simulink model "Kalman_filter"  (R2025b)
settings: Solver=FixedStepAuto  StartTime=0.0  StopTime=20  FixedStep=0.002  RelTol=1e-3
values from neighbouring files (symbols this model uses):
  A_pitch = [X_hat_u  X_hat_q   g  0 ... (first row only)    [Parameters.m]
  A_py = blkdiag(A_pitch, A_yaw)    [Parameters.m]
  A_yaw = [N_hat_r  1/I_zz ... (first row only)    [Parameters.m]
  B_py = blkdiag(B_pitch, B_yaw)    [Parameters.m]
  C_pitch = [X_hat_u+d_new*M_hat_u  X_hat_q+d_new*M_hat_q   0   d_new/I_yy;      0        1           0   0]    [Parameters.m]
  C_py = blkdiag(C_pitch, C_yaw)    [Parameters.m]
  C_yaw = [1   0]    [Parameters.m]
  k_r = 0.8e-5    (= 8e-06)    [Parameters.m]
  kd_p = 0.27*kth_p    (= 0.0005184)    [Parameters.m]
  kth_p = 192e-5    (= 0.00192)    [Parameters.m]
  L_ob_py = X1_py*C_py'*(R_n_py^-1)    [Parameters.m]
  LC_DEN = [1 p1]    [Parameters.m]
  LC_NUM = gain*(p1/z1)*[1 z1]    [Parameters.m]
  T_psi = 0.15    [Parameters.m]
  u_gain = -X_hat_u/g    (= 0.0967315158219)    [Parameters.m]
  x_hat_py = [0 0 0 0 0 0]'    [Parameters.m]
  x_pitch = [0.1 0 2*pi/180 0]'    [Parameters.m]
  x_yaw = [5*pi/180 2*pi/180 0]'    [Parameters.m]
libraries: slpidlib x2
settings Model: Creator=yfari  LastModifiedBy=yfari
settings OptimizationCC: ReuseModelBlockBuffer=off
settings DebuggingCC: UnconnectedInputMsg=warning  UnconnectedOutputMsg=warning  UnconnectedLineMsg=warning
settings ModelReferenceCC: EnableRefExpFcnMdlSchedulingChecks=on
settings RTWCC: GPUComputeCapability=3.5  DLArmComputeVersion=19.05

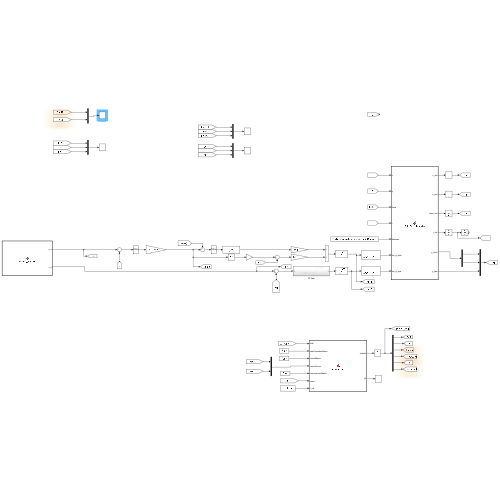
[thumbnail: Simulink's stored preview of the top-level diagram]
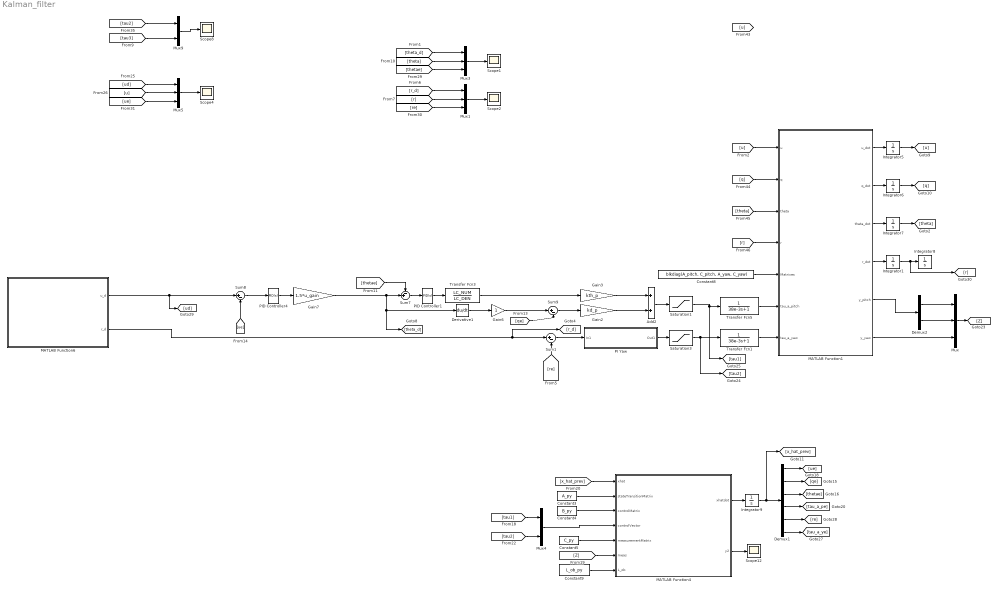
== system Kalman_filter ==
  Add2 : Sum
  Constant3 : Constant  Value=A_py
  Constant4 : Constant  Value=B_py
  Constant5 : Constant  Value=C_py
  Constant8 : Constant  Value=blkdiag(A_pitch, C_pitch, A_yaw, C_yaw)  VectorParams1D=off
  Constant9 : Constant  Value=L_ob_py
  Demux1 : Demux  Outputs=6
  Demux2 : Demux  Outputs=2
  Derivative1 : Derivative
  Gain2 : Gain  Gain=kd_p
  Gain3 : Gain  Gain=kth_p
  Gain6 : Gain
  Gain7 : Gain  Gain=1.5*u_gain
  Integrator1 : Integrator  InitialCondition=x_yaw(1)
  Integrator5 : Integrator  InitialCondition=x_pitch(1)
  Integrator6 : Integrator  InitialCondition=x_pitch(2)
  Integrator7 : Integrator  InitialCondition=x_pitch(3)
  Integrator8 : Integrator  InitialCondition=0*pi/180
  Integrator9 : Integrator  InitialCondition=x_hat_py
  MATLAB Function1 : MATLAB Function  TreatAsAtomicUnit=on
  MATLAB Function4 : MATLAB Function  TreatAsAtomicUnit=on
  MATLAB Function6 : MATLAB Function  TreatAsAtomicUnit=on
  Mux{,1,3,5} (4 alike) : Mux  Inputs=3
  Mux4 : Mux  Inputs=2
  Mux9 : Mux  Inputs=2
  PI Yaw : Subsystem
  PID Controller1 : slpidlib/PID Controller  Controller=PID  Form=Ideal  TimeDomain=Continuous-time  UseExternalTs=off  SampleTime=-1  IntegratorMethod=Forward Euler  FilterMethod=Forward Euler  ControllerParametersSource=internal  P=1  I=2*pi*0.2  UseKiTs=off  D=0  UseExternalDerivativeSource=off  N=100  UseFilter=on  TunerSelectOption=Transfer Function Based (PID Tuner App)  InitialConditionSource=internal  InitialConditionForIntegrator=0  InitialConditionForFilter=0  DifferentiatorICPrevScaledInput=0  ExternalReset=none  TrackingMode=off  Kt=1  LimitOutput=off  SatLimitsSource=internal  UpperSaturationLimit=inf  LowerSaturationLimit=-inf  LinearizeAsGain=on  AntiWindupMode=none  Kb=1  LimitIntegrator=off  UpperIntegratorSaturationLimit=inf  LowerIntegratorSaturationLimit=-inf  POutMin=[]  POutMax=[]  IOutMin=[]  IOutMax=[]  DOutMin=[]  DOutMax=[]  NOutMin=[]  NOutMax=[]  SumOutMin=[]  SumOutMax=[]  SaturationOutMin=[]  SaturationOutMax=[]  PParamMin=[]  PParamMax=[]  IParamMin=[]  IParamMax=[]  DParamMin=[]  DParamMax=[]  NParamMin=[]  NParamMax=[]  KbParamMin=[]  KbParamMax=[]  KtParamMin=[]  KtParamMax=[]  KbOutMin=[]  KbOutMax=[]  KtOutMin=[]  KtOutMax=[]  IntegratorOutMin=[]  IntegratorOutMax=[]  FilterOutMin=[]  FilterOutMax=[]  SumI1OutMin=[]  SumI1OutMax=[]  SumI2OutMin=[]  SumI2OutMax=[]  SumI3OutMin=[]  SumI3OutMax=[]  SumI4OutMin=[]  SumI4OutMax=[]  SumDOutMin=[]  SumDOutMax=[]  DifferentiatorOutMin=[]  DifferentiatorOutMax=[]  FilterDiffOutCoefMin=[]  FilterDiffOutCoefMax=[]  ReciprocalOutMin=[]  ReciprocalOutMax=[]  SumDenOutMin=[]  SumDenOutMax=[]  SumNumOutMin=[]  SumNumOutMax=[]  DivideOutMin=[]  DivideOutMax=[]  UdiffTsProdOutMin=[]  UdiffTsProdOutMax=[]  NTsProdOutMin=[]  NTsProdOutMax=[]  UintegralTsProdOutMin=[]  UintegralTsProdOutMax=[]  UngainTsProdOutMin=[]  UngainTsProdOutMax=[]  ClampingZeroOutDataTypeStr=Inherit: Inherit via back propagation  ClampingZeroOutMin=[]  ClampingZeroOutMax=[]  FilterDenConstantOutDataTypeStr=Inherit: Inherit via back propagation  FilterDenConstantOutMin=[]  FilterDenConstantOutMax=[]  PCopyOutDataTypeStr=Inherit: Inherit via back propagation  PCopyOutMin=[]  PCopyOutMax=[]  NCopyOutDataTypeStr=Inherit: Inherit via back propagation  NCopyOutMin=[]  NCopyOutMax=[]  IntegratorContinuousStateAttributes=''  IntegratorStateMustResolveToSignalObject=off  IntegratorRTWStateStorageClass=Auto  FilterContinuousStateAttributes=''  FilterStateMustResolveToSignalObject=off  FilterRTWStateStorageClass=Auto  ParallelPVariant=Passthrough  IdealPVariant=InternalParameters  IVariant=InternalParameters  DVariant=InternalParameters  IntegratorVariant=Continuous  SatVariant=Disabled  AWVariant=Passthrough  PCopyVariant=Disabled  TRVariant=Disabled  FdbkBlocksVariant=Forward  IdealPFdbkVariant=Disabled  SatFdbkVariant=Disabled  DerivativeFilterVariant=ContFilter  NVariant=InternalParameters  NCopyVariant=Disabled  FilterICVariant=InternalICsFilter  IntegratorICVariant=InternalICs  ExternalResetVariant=Disabled  TRSumVariant=Passthrough  SumFdbkVariant=Disabled  SumVariant=Sum_PID  TsampFilterVariant=InternalTs  TsampNgainVariant=Passthrough  TsampIntegralVariant=Disabled_SignalSpec  ExternalSaturationOutDataTypeStr=Inherit: Same as second input  DerivativeSourceVariant=ErrorSignal  PreIntVariant=InternalPreInt
  PID Controller4 : slpidlib/PID Controller  Controller=PID  Form=Ideal  TimeDomain=Continuous-time  UseExternalTs=off  SampleTime=-1  IntegratorMethod=Forward Euler  FilterMethod=Forward Euler  ControllerParametersSource=internal  P=1  I=2  UseKiTs=off  D=0  UseExternalDerivativeSource=off  N=100  UseFilter=on  TunerSelectOption=Transfer Function Based (PID Tuner App)  InitialConditionSource=internal  InitialConditionForIntegrator=0  InitialConditionForFilter=0  DifferentiatorICPrevScaledInput=0  ExternalReset=none  TrackingMode=off  Kt=1  LimitOutput=off  SatLimitsSource=internal  UpperSaturationLimit=inf  LowerSaturationLimit=-inf  LinearizeAsGain=on  AntiWindupMode=none  Kb=1  LimitIntegrator=off  UpperIntegratorSaturationLimit=inf  LowerIntegratorSaturationLimit=-inf  POutMin=[]  POutMax=[]  IOutMin=[]  IOutMax=[]  DOutMin=[]  DOutMax=[]  NOutMin=[]  NOutMax=[]  SumOutMin=[]  SumOutMax=[]  SaturationOutMin=[]  SaturationOutMax=[]  PParamMin=[]  PParamMax=[]  IParamMin=[]  IParamMax=[]  DParamMin=[]  DParamMax=[]  NParamMin=[]  NParamMax=[]  KbParamMin=[]  KbParamMax=[]  KtParamMin=[]  KtParamMax=[]  KbOutMin=[]  KbOutMax=[]  KtOutMin=[]  KtOutMax=[]  IntegratorOutMin=[]  IntegratorOutMax=[]  FilterOutMin=[]  FilterOutMax=[]  SumI1OutMin=[]  SumI1OutMax=[]  SumI2OutMin=[]  SumI2OutMax=[]  SumI3OutMin=[]  SumI3OutMax=[]  SumI4OutMin=[]  SumI4OutMax=[]  SumDOutMin=[]  SumDOutMax=[]  DifferentiatorOutMin=[]  DifferentiatorOutMax=[]  FilterDiffOutCoefMin=[]  FilterDiffOutCoefMax=[]  ReciprocalOutMin=[]  ReciprocalOutMax=[]  SumDenOutMin=[]  SumDenOutMax=[]  SumNumOutMin=[]  SumNumOutMax=[]  DivideOutMin=[]  DivideOutMax=[]  UdiffTsProdOutMin=[]  UdiffTsProdOutMax=[]  NTsProdOutMin=[]  NTsProdOutMax=[]  UintegralTsProdOutMin=[]  UintegralTsProdOutMax=[]  UngainTsProdOutMin=[]  UngainTsProdOutMax=[]  ClampingZeroOutDataTypeStr=Inherit: Inherit via back propagation  ClampingZeroOutMin=[]  ClampingZeroOutMax=[]  FilterDenConstantOutDataTypeStr=Inherit: Inherit via back propagation  FilterDenConstantOutMin=[]  FilterDenConstantOutMax=[]  PCopyOutDataTypeStr=Inherit: Inherit via back propagation  PCopyOutMin=[]  PCopyOutMax=[]  NCopyOutDataTypeStr=Inherit: Inherit via back propagation  NCopyOutMin=[]  NCopyOutMax=[]  IntegratorContinuousStateAttributes=''  IntegratorStateMustResolveToSignalObject=off  IntegratorRTWStateStorageClass=Auto  FilterContinuousStateAttributes=''  FilterStateMustResolveToSignalObject=off  FilterRTWStateStorageClass=Auto  ParallelPVariant=Passthrough  IdealPVariant=InternalParameters  IVariant=InternalParameters  DVariant=InternalParameters  IntegratorVariant=Continuous  SatVariant=Disabled  AWVariant=Passthrough  PCopyVariant=Disabled  TRVariant=Disabled  FdbkBlocksVariant=Forward  IdealPFdbkVariant=Disabled  SatFdbkVariant=Disabled  DerivativeFilterVariant=ContFilter  NVariant=InternalParameters  NCopyVariant=Disabled  FilterICVariant=InternalICsFilter  IntegratorICVariant=InternalICs  ExternalResetVariant=Disabled  TRSumVariant=Passthrough  SumFdbkVariant=Disabled  SumVariant=Sum_PID  TsampFilterVariant=InternalTs  TsampNgainVariant=Passthrough  TsampIntegralVariant=Disabled_SignalSpec  ExternalSaturationOutDataTypeStr=Inherit: Same as second input  DerivativeSourceVariant=ErrorSignal  PreIntVariant=InternalPreInt
  Saturation1 : Saturate  UpperLimit=0.002  LowerLimit=-0.002
  Saturation3 : Saturate  UpperLimit=0.002  LowerLimit=-0.002
  Scope{1..2,4,8,12} (5 alike) : Scope
      Scope1 settings: ActiveDisplayYMinimum=-0.024055899110475627  ActiveDisplayYMaximum=0.21650309199428069
      Scope12 settings: ActiveDisplayYMinimum=-1  ActiveDisplayYMaximum=1  DataLoggingVariableName=ScopeData8
      Scope2 settings: ActiveDisplayYMinimum=-0.12499999999999997  ActiveDisplayYMaximum=1.125  DataLoggingVariableName=ScopeData12
      Scope4 settings: ActiveDisplayYMinimum=-1.7486026491281286  ActiveDisplayYMaximum=0.82715164299244548  DataLoggingVariableName=ScopeData2
      Scope8 settings: ActiveDisplayYMinimum=-0.02276  ActiveDisplayYMaximum=0.02375  DataLoggingVariableName=ScopeData4
  Sum1 : Sum  Inputs=|+-
  Sum7 : Sum  Inputs=-+|
  Sum8 : Sum  Inputs=|+-
  Sum9 : Sum  Inputs=|+-
  Transfer Fcn1 : TransferFcn  Denominator=[38e-3 1]
  Transfer Fcn3 : TransferFcn  Numerator=LC_NUM  Denominator=LC_DEN
  Transfer Fcn5 : TransferFcn  Denominator=[38e-3 1]
  wires:
  Mux3/1 -> Scope1/1
  PID Controller4/1 -> Gain7/1
  MATLAB Function1/2(q_dot) -> Integrator6/1
  MATLAB Function4/2(y2) -> Scope12/1
  Integrator6/1 -> [q]
  [theta_d] -> Mux3/1
  [re] -> Mux1/3
  Mux4/1 -> MATLAB Function4/4(controlVector)
  [r] -> MATLAB Function1/4(r)
  Transfer Fcn3/1 -> Gain3/1
  Constant8/1 -> MATLAB Function1/5(Matrixes)
  [q] -> MATLAB Function1/2(q)
  Gain7/1 -> Sum7/2, [theta_d], Derivative1/1
  [r] -> Mux1/2
  Sum7/1 -> PID Controller1/1
  Integrator9/1 -> [x_hat_prev], Demux1/1
  Transfer Fcn5/1 -> MATLAB Function1/6(tau_a_pitch)
  MATLAB Function4/1(xhatdot) -> Integrator9/1
  Mux5/1 -> Scope4/1
  Constant5/1 -> MATLAB Function4/5(measurementMatrix)
  Mux9/1 -> Scope8/1
  [thetae] -> Mux3/3
  Integrator7/1 -> [theta]
  MATLAB Function1/1(u_dot) -> Integrator5/1
  PID Controller1/1 -> Transfer Fcn3/1
  [x_hat_prev] -> MATLAB Function4/1(xhat)
  [ue] -> Mux5/3
  [ud] -> Mux5/1
  [Z] -> MATLAB Function4/6(meas)
  Gain3/1 -> Add2/1
  [r_d] -> Mux1/1
  [u] -> Mux5/2
  MATLAB Function6/2(r_d) -> [r_d], Sum1/1
  Derivative1/1 -> Gain6/1
  MATLAB Function1/4(r_dot) -> Integrator1/1
  Constant9/1 -> MATLAB Function4/7(L_ob)
  [theta] -> MATLAB Function1/3(theta)
  Mux/1 -> [Z]
  Mux1/1 -> Scope2/1
  Integrator5/1 -> [u]
  MATLAB Function6/1(u_d) -> [ud], Sum8/1
  MATLAB Function1/3(theta_dot) -> Integrator7/1
  [qe] -> Sum9/2
  [theta] -> Mux3/2
  Integrator1/1 -> [r], Integrator8/1
  Constant3/1 -> MATLAB Function4/2(stateTransitionMatrix)
  Gain2/1 -> Add2/2
  Gain6/1 -> Sum9/1
  Transfer Fcn1/1 -> MATLAB Function1/7(tau_a_yaw)
  Constant4/1 -> MATLAB Function4/3(controlMatrix)
  [thetae] -> Sum7/1
  [ue] -> Sum8/2
  Sum1/1 -> PI Yaw/1(In1)
  Sum9/1 -> Gain2/1
  [re] -> Sum1/2
  Sum8/1 -> PID Controller4/1
  PI Yaw/1(Out1) -> Saturation3/1
  Add2/1 -> Saturation1/1
  Saturation1/1 -> [tau1], Transfer Fcn5/1
  Saturation3/1 -> [tau2], Transfer Fcn1/1
  [tau2] -> Mux9/1
  [tau3] -> Mux9/2
  [u] -> MATLAB Function1/1(u)
  MATLAB Function1/6(y_yaw) -> Mux/3
  Demux2/2 -> Mux/2
  Demux2/1 -> Mux/1
  MATLAB Function1/5(y_pitch) -> Demux2/1
  Demux1/1 -> [ue]
  Demux1/2 -> [qe]
  Demux1/3 -> [thetae]
  Demux1/4 -> [tau_a_pe]
  Demux1/5 -> [re]
  Demux1/6 -> [tau_a_ye]
  [tau2] -> Mux4/2
  [tau1] -> Mux4/1

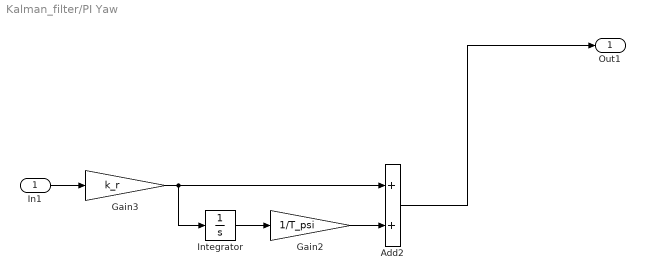
== system Kalman_filter/PI Yaw ==
  In1 : Inport
  Add2 : Sum
  Gain2 : Gain  Gain=1/T_psi
  Gain3 : Gain  Gain=k_r
  Integrator : Integrator
  Out1 : Outport
  wires:
  Add2/1 -> Out1/1
  Gain2/1 -> Add2/2
  Gain3/1 -> Integrator/1, Add2/1
  In1/1 -> Gain3/1
  Integrator/1 -> Gain2/1

== matlab function Kalman_filter/MATLAB Function1 ==
  data: u input; u_dot output; q input; theta input; r input; Matrixes input; q_dot output; theta_dot output; r_dot output; tau_a_pitch input; y_pitch output; y_yaw output; tau_a_yaw input
function [u_dot, q_dot, theta_dot, r_dot,y_pitch, y_yaw] = Roll_Pitch_dynamics(u, q, theta, r, Matrixes, tau_a_pitch, tau_a_yaw)

A_pitch = Matrixes(1:4,  1:4);
C_pitch = Matrixes(5:6,  5:8);
A_yaw = Matrixes(7:8,  9:10);
C_yaw = Matrixes(9,  11:12);

%% pitch dynamics
X_pitch = [u, q, theta, tau_a_pitch]';
Xdot_pitch = A_pitch(1:3,:) * X_pitch;
u_dot = Xdot_pitch(1);
q_dot = Xdot_pitch(2);
theta_dot  = Xdot_pitch(3);
%% yaw dynamics
X_yaw = [r, tau_a_yaw]';
Xdot_yaw = A_yaw(1:1,:) * X_yaw;
r_dot = Xdot_yaw(1);
%% Measurements
y_pitch = C_pitch * X_pitch;
y_yaw   = C_yaw * X_yaw;

== matlab function Kalman_filter/MATLAB Function4 ==
  data: xhatdot output; xhat input; stateTransitionMatrix input; controlMatrix input; controlVector input; measurementMatrix input; meas input; L_ob input; y2 output
function [xhatdot, y2]  = kalman_filter(xhat,stateTransitionMatrix,controlMatrix,controlVector, measurementMatrix,meas,L_ob)

A = stateTransitionMatrix;
B = controlMatrix;
u = controlVector;
C = measurementMatrix;

% calculate the residual
residual = meas - C*xhat;

xhatdot = A*xhat + B*u + L_ob*residual;
y2 = residual;

end

== matlab function Kalman_filter/MATLAB Function6 ==
  data: u_d output; r_d output
function [u_d, r_d] = circular_outputs

u_d = 1; 
%% yaw rate
r_d = 1; 

end
